simulink model "MUTfinal2"  (R2022b)
settings: Solver=VariableStepAuto  StartTime=0.0  StopTime=tFinal  RelTol=1e-3
values from neighbouring files (symbols this model uses):
  C1 = C1_OLD    [DPP_PSO.m]    (also in PlotEvaluateResponse.m = 1.59e-06)
  C2 = C2_OLD    [DPP_PSO.m]    (also in PlotEvaluateResponse.m = 1.59e-06)
  Cn = Cn_OLD    [DPP_PSO.m]    (also in PlotEvaluateResponse.m = 7.95e-07)
  F = 20e3    (= 20000)    [DPP_PSO.m]    (also in PlotEvaluateResponse.m)
  G1 = 1000    [DPP_PSO.m]    (also in PlotEvaluateResponse.m)
  L1 = L1_OLD    [DPP_PSO.m]    (also in PlotEvaluateResponse.m = 0.0049)
  L2 = L2_OLD    [DPP_PSO.m]    (also in PlotEvaluateResponse.m = 0.0049)
  sample_time = 1e-6    (= 1e-06)    [DPP_PSO.m]    (also in PlotEvaluateResponse.m)
  VBus = 36    [DPP_PSO.m]    (also in PlotEvaluateResponse.m)
undefined symbols (not defined in the file or in its folder): sigbuilder_block
libraries: spsSeriesRLCBranchLib x6, spsCurrentMeasurementLib x6, spsVoltageMeasurementLib x4, spsDiodeLib x2, spsPVArrayLib x2, spsMosfetLib x2, spsDCVoltageSourceLib x1, spspowerguiLib x1
settings Model: Creator=gta12345_v  LastModifiedBy=AEssa
settings ModelReferenceCC: EnableRefExpFcnMdlSchedulingChecks=on

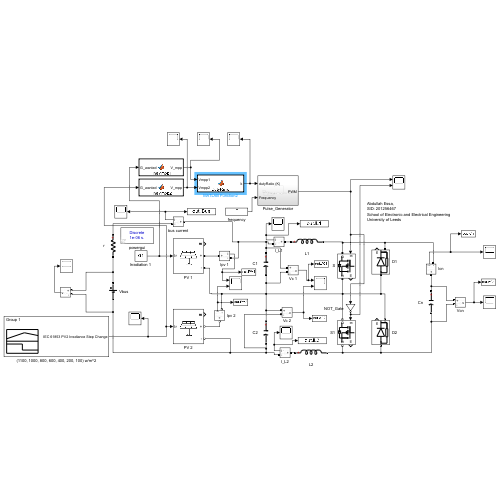
[thumbnail: Simulink's stored preview of the top-level diagram]
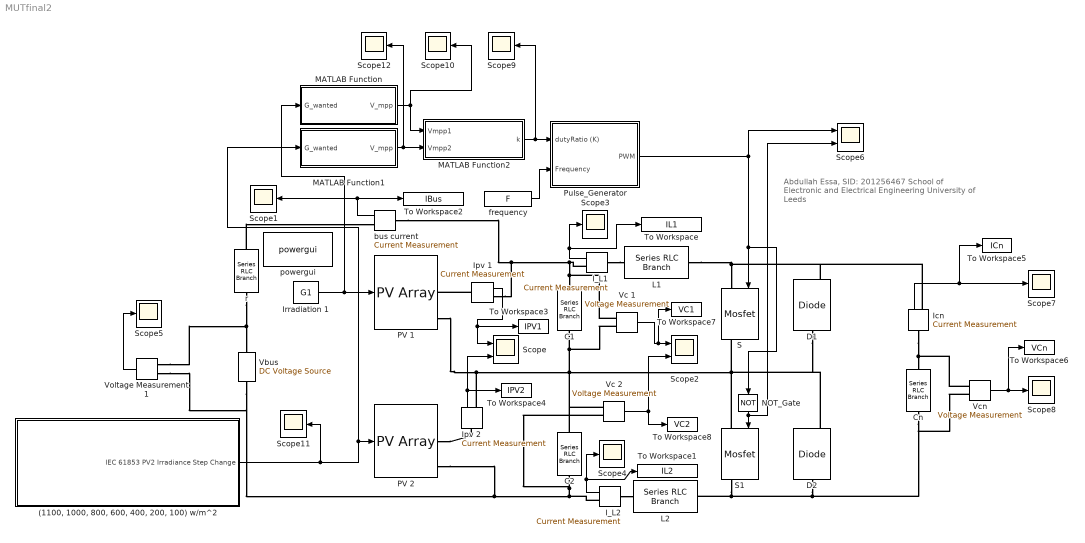
== system MUTfinal2 ==
  note: Abdullah Essa,
      | SID: 201256467
      | School of Electronic and Electrical Engineering
      | University of Leeds
  "(1100, 1000, 800, 600, 400, 200, 100) w/m^2" : Subsystem  Tag=STV Subsys  LoadFcn=sigbuilder_block('load');  StartFcn=sigbuilder_block('start');  StopFcn=sigbuilder_block('stop');  ClipboardFcn=sigbuilder_block('clipboard');  mask(Sigbuilder block){tuvar=[0:10]}
      mask help: Simulink:masks:SigbuilderBlock_MD
      mask init:
      | if ~strcmp(get_param(bdroot(gcbh),'SimulationStatus'),'stopped') tuvar = sigbuilder_block('maskInit'); end
      settings: CopyFcn=sigbuilder_block('copy');  DeleteFcn=sigbuilder_block('delete');  ModelCloseFcn=sigbuilder_block('modelClose');  PreSaveFcn=sigbuilder_block('preSave');  PauseFcn=sigbuilder_block('pause');  ContinueFcn=sigbuilder_block('continue');  NameChangeFcn=sigbuilder_block('namechange');  OpenFcn=sigbuilder_block('open',[420 17.25 550.5 399.75 ]);  CloseFcn=sigbuilder_block('close');
      mask Display: plot(0, 0, 100, 100,[2, 2, 32, 32, 2], [68, 8, 8, 68, 68],[32, 2], [38, 38], [32, 19, 2],[53, 60, 44], [32, 17, 17, 2],[16, 16, 31, 31]);txt = getActiveGroup(gcbh);text(2, 100, txt,'verticalAlignment', 'top');
  C1 : spsSeriesRLCBranchLib/Series RLC Branch  LConnTagsString=__new0  RConnTagsString=__new0  BranchType=C  Resistance=1  Inductance=1e-3  SetiL0=off  InitialCurrent=0  Capacitance=C1  Setx0=off  InitialVoltage=0  Measurements=None
  C2 : spsSeriesRLCBranchLib/Series RLC Branch  LConnTagsString=__new0  RConnTagsString=__new0  BranchType=C  Resistance=1  Inductance=1e-3  SetiL0=off  InitialCurrent=0  Capacitance=C2  Setx0=off  InitialVoltage=0  Measurements=None
  Cn : spsSeriesRLCBranchLib/Series RLC Branch  LConnTagsString=__new0  RConnTagsString=__new0  BranchType=C  Resistance=1  Inductance=1e-3  SetiL0=off  InitialCurrent=0  Capacitance=Cn  Setx0=off  InitialVoltage=0  Measurements=None
  D1 : spsDiodeLib/Diode  Ron=0.001  Lon=0  Vf=0.8  IC=0  UseSnubber=0  Rs=500  Cs=250e-9  Measurements=on
  D2 : spsDiodeLib/Diode  Ron=0.001  Lon=0  Vf=0.8  IC=0  UseSnubber=0  Rs=500  Cs=250e-9  Measurements=on
  I_L1 : spsCurrentMeasurementLib/Current Measurement  PhasorSimulation=off  OutputType=Complex  PSBequivalent=0
  I_L2 : spsCurrentMeasurementLib/Current Measurement  PhasorSimulation=off  OutputType=Complex  PSBequivalent=0
  "Icn " : spsCurrentMeasurementLib/Current Measurement  PhasorSimulation=off  OutputType=Complex  PSBequivalent=0
  Ipv 1 : spsCurrentMeasurementLib/Current Measurement  PhasorSimulation=off  OutputType=Complex  PSBequivalent=0
  Ipv 2 : spsCurrentMeasurementLib/Current Measurement  PhasorSimulation=off  OutputType=Complex  PSBequivalent=0
  "Irradiation 1 " : Constant  Value=G1  SampleTime=Inf
  L1 : spsSeriesRLCBranchLib/Series RLC Branch  LConnTagsString=__new0  RConnTagsString=__new0  BranchType=L  Resistance=1  Inductance=L1  SetiL0=off  InitialCurrent=0  Capacitance=1e-6  Setx0=off  InitialVoltage=0  Measurements=None
  L2 : spsSeriesRLCBranchLib/Series RLC Branch  LConnTagsString=__new0  RConnTagsString=__new0  BranchType=L  Resistance=1  Inductance=L2  SetiL0=off  InitialCurrent=0  Capacitance=1e-6  Setx0=off  InitialVoltage=0  Measurements=None
  MATLAB Function : MATLAB Function  TreatAsAtomicUnit=on
  MATLAB Function1 : MATLAB Function  TreatAsAtomicUnit=on
  MATLAB Function2 : MATLAB Function  TreatAsAtomicUnit=on
  NOT_Gate : Logic  Operator=NOT  IconShape=distinctive  AllPortsSameDT=off  OutDataTypeStr=boolean
  PV 1 : spsPVArrayLib/PV Array  Npar=1  Nser=1  PlotType=one module @ 25 deg.C & specified irradiances  S_vec="[ 1000  500  100 ]"  Temp_C_vec="[ 45 25  ]"  ModuleName=Canadian Solar Inc. CS5C-90M  PlotWhenSelected=off  Pm=89.82  Ncell=36  Voc=22.2  Isc=5.4  Vm=18  Im=4.99  beta_Voc_pc=-0.374  alpha_Isc_pc=0.089  beta_Voc=-0.083028  alpha_Isc=0.004806  IL=5.4115  I0=3.0531e-10  nI=1.0185  Rsh=134.0722  Rs=0.2862  RobustModel=on  RobustCellTemperature=25  BAL=on  Tc=1e-6  Tfilter=5e-5
  PV 2 : spsPVArrayLib/PV Array  Npar=1  Nser=1  PlotType=one module @ 25 deg.C & specified irradiances  S_vec="[ 1000  500  100 ]"  Temp_C_vec="[ 45 25  ]"  ModuleName=Canadian Solar Inc. CS5C-90M  PlotWhenSelected=off  Pm=89.82  Ncell=36  Voc=22.2  Isc=5.4  Vm=18  Im=4.99  beta_Voc_pc=-0.374  alpha_Isc_pc=0.089  beta_Voc=-0.083028  alpha_Isc=0.004806  IL=5.4115  I0=3.0531e-10  nI=1.0185  Rsh=134.0722  Rs=0.2862  RobustModel=on  RobustCellTemperature=25  BAL=on  Tc=1e-6  Tfilter=5e-5
  Pulse_Generator : Subsystem
  S : spsMosfetLib/Mosfet  Ron=0.1  Lon=0  Rd=0.01  Vfd=0  IC=0  Rs=1e5  Cs=inf  Measurements=on
  S1 : spsMosfetLib/Mosfet  Ron=0.1  Lon=0  Rd=0.01  Vfd=0  IC=0  Rs=1e5  Cs=inf  Measurements=on
  Scope : Scope  NumInputPorts=2
  Scope{1,3..5,7..12} (10 alike) : Scope
  Scope2 : Scope  NumInputPorts=2
  Scope6 : Scope  NumInputPorts=2
  To Workspace : ToWorkspace  VariableName=IL1  SaveFormat=Timeseries  SampleTime=-1
  To Workspace1 : ToWorkspace  VariableName=IL2  SaveFormat=Timeseries  SampleTime=-1
  To Workspace2 : ToWorkspace  VariableName=IBus  SaveFormat=Timeseries  SampleTime=-1
  To Workspace3 : ToWorkspace  VariableName=IPV1  SaveFormat=Timeseries  SampleTime=-1
  To Workspace4 : ToWorkspace  VariableName=IPV2  SaveFormat=Timeseries  SampleTime=-1
  To Workspace5 : ToWorkspace  VariableName=ICn  SaveFormat=Timeseries  SampleTime=-1
  To Workspace6 : ToWorkspace  VariableName=VCn  SaveFormat=Timeseries  SampleTime=-1
  To Workspace7 : ToWorkspace  VariableName=VC1  SaveFormat=Timeseries  SampleTime=-1
  To Workspace8 : ToWorkspace  VariableName=VC2  SaveFormat=Timeseries  SampleTime=-1
  Vbus : spsDCVoltageSourceLib/DC Voltage Source  Amplitude=VBus  Measurements=None
  Vc 1 : spsVoltageMeasurementLib/Voltage Measurement  PhasorSimulation=off  OutputType=Complex  PSBequivalent=0
  Vc 2 : spsVoltageMeasurementLib/Voltage Measurement  PhasorSimulation=off  OutputType=Complex  PSBequivalent=0
  Vcn : spsVoltageMeasurementLib/Voltage Measurement  PhasorSimulation=off  OutputType=Complex  PSBequivalent=0
  Voltage Measurement1 : spsVoltageMeasurementLib/Voltage Measurement  PhasorSimulation=off  OutputType=Complex  PSBequivalent=0
  bus current : spsCurrentMeasurementLib/Current Measurement  PhasorSimulation=off  OutputType=Complex  PSBequivalent=0
  frequency : Constant  Value=F
  powergui : spspowerguiLib/powergui  Priority=1  SimulationMode=Discrete  SampleTime=sample_time  frequency=60  Iterations=50  frequencyindice=0  Pbase=100e6  ErrMax=1e-4  UnitsV=kV  UnitsW=MW  buscounter=0  FunctionMessages=off  echomessages=off  EnableUseOfTLC=off  CurrentSourceSwitches=off  DisableSnubberDevices=off  DisableRonSwitches=off  DisableVfSwitches=off  DisplayEquations=off  AutomaticDiscreteSolvers=off  SolverType=Tustin/Backward Euler (TBE)  Interpol=off  ExternalGateDelay=off  methode=off  Ts=100  x0status=blocks  SPID=on  SwTol=0  HookPort=off  NonlinearTolerance=1e-4  nMaxIteration=100  ContinueOnMaxIteration=off  RestoreLinks=warning  ResistiveCurrentMeasurement=off  Frange=[0:2:500]  Ylog=off  Xlog=on  ShowGrid=off  save=off  variable=ZData  structure=0  ZoomFFT=off  StartTime=0.0  cycles=1  DisplayStyle=1  fundamental=60  FreqAxis=off  MaxFrequency=1000  frequencyindicesteady=1  RmsSteady=1  display=off
  r : spsSeriesRLCBranchLib/Series RLC Branch  LConnTagsString=__new0  RConnTagsString=__new0  BranchType=R  Resistance=0.1  Inductance=1e-3  SetiL0=off  InitialCurrent=0  Capacitance=1.59e-6  Setx0=off  InitialVoltage=0  Measurements=None
  wires:
  "Irradiation 1 "/1 -> MATLAB Function/1(G_wanted), PV 1/1
  Pulse_Generator/1(PWM) -> Scope6/1, NOT_Gate/1, S/1
  NOT_Gate/1 -> Scope6/2, S1/1
  Ipv 2/1 -> To Workspace4/1, Scope/2
  Ipv 1/1 -> To Workspace3/1, Scope/1
  bus current/1 -> To Workspace2/1, Scope1/1
  Vc 1/1 -> To Workspace7/1, Scope2/1
  I_L2/1 -> Scope4/1, To Workspace1/1
  I_L1/1 -> To Workspace/1, Scope3/1
  Voltage Measurement1/1 -> Scope5/1
  "(1100, 1000, 800, 600, 400, 200, 100) w/m^2"/1(IEC 61853 PV2 Irradiance Step Change) -> Scope11/1, MATLAB Function1/1(G_wanted), PV 2/1
  frequency/1 -> Pulse_Generator/2(Frequency)
  Vc 2/1 -> To Workspace8/1, Scope2/2
  "Icn "/1 -> To Workspace5/1, Scope7/1
  Vcn/1 -> To Workspace6/1, Scope8/1
  MATLAB Function/1(V_mpp) -> MATLAB Function2/1(Vmpp1), Scope10/1
  MATLAB Function1/1(V_mpp) -> Scope12/1, MATLAB Function2/2(Vmpp2)
  MATLAB Function2/1(k) -> Scope9/1, Pulse_Generator/1(dutyRatio (K))
  connections:
  bus current/LConn1 -- Ipv 1/RConn1 -- Vc 1/LConn1 -- C1/LConn1 -- I_L1/RConn1
  PV 2/RConn2 -- Vbus/LConn1 -- Voltage Measurement1/LConn2 -- I_L2/RConn1 -- Vc 2/LConn2 -- C2/RConn1
  L1/RConn1 -- "Icn "/RConn1 -- D1/RConn1 -- S/LConn1
  PV 1/RConn2 -- Ipv 2/RConn1 -- Vc 2/LConn1 -- C2/LConn1 -- Vc 1/LConn2 -- C1/RConn1 -- D2/RConn1 -- D1/LConn1 -- S/RConn1 -- S1/LConn1
  S1/RConn1 -- Vcn/LConn2 -- Cn/RConn1 -- D2/LConn1 -- L2/RConn1
  Voltage Measurement1/LConn1 -- r/RConn1 -- Vbus/RConn1
  Ipv 1/LConn1 -- PV 1/RConn1
  PV 2/RConn1 -- Ipv 2/LConn1
  I_L1/LConn1 -- L1/LConn1
  I_L2/LConn1 -- L2/LConn1
  r/LConn1 -- bus current/RConn1
  "Icn "/LConn1 -- Vcn/LConn1 -- Cn/LConn1

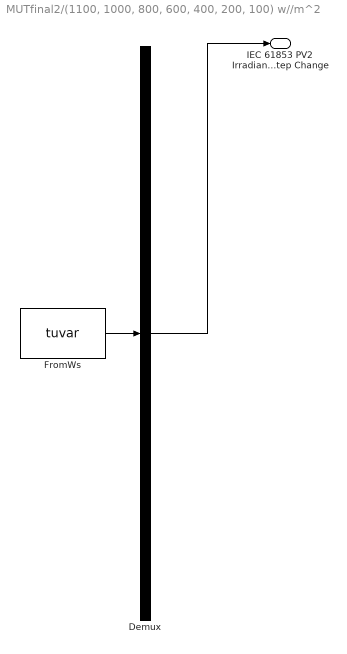
== system MUTfinal2/(1100, 1000, 800, 600, 400, 200, 100) w//m^2 ==
  Demux : Demux  Tag=STV Demux  Outputs=1
      settings: DisplayOption=none
  FromWs : FromWorkspace  Tag=STV FromWs  VariableName=tuvar
      SigBuilderData=|
      | common.afterFinalStr = 'Extrapolate'
      | common.sampleTime = 0
      | dataSet.timeRange = [0 0.14]
      | dataSet.name = 'Group 1'
      | sbobj.Groups.Name = 'Group 1'
      | sbobj.Groups.Signals.Name = 'IEC 61853 PV2 Irradiance Step Change'
      | sbobj.Groups.Signals.XData = [0 0.02 0.02 0.04 0.04 0.06 0.06 0.08 0.08 0.1 0.1 0.12 0.12 0.14]
      | sbobj.Groups.Signals.YData = [1100 1100 1000 1000 800 800 600 600 400 400 200 200 100 100]
      | sbobj.Groups.TimeRange = [0 0.14]
  IEC 61853 PV2 Irradiance Step Change : Outport  Tag=STV Outport
  wires:
  Demux/1 -> IEC 61853 PV2 Irradiance Step Change/1
  FromWs/1 -> Demux/1

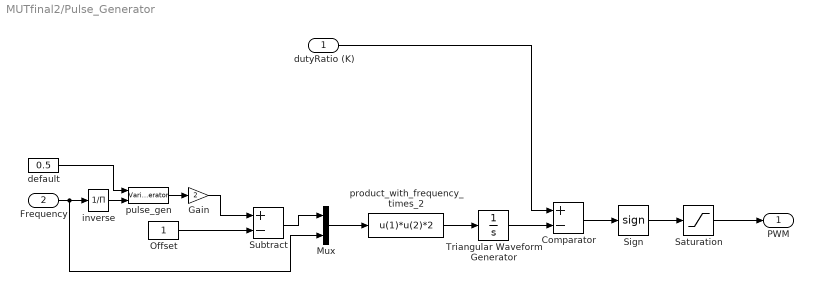
== system MUTfinal2/Pulse_Generator ==
  dutyRatio (K) : Inport
  Frequency : Inport  Port=2
  Comparator : Sum  Inputs=+-
  Gain : Gain  Gain=2
  Mux : Mux  Inputs=2
  Offset : Constant
  Saturation : Saturate  UpperLimit=1  LowerLimit=0
  Sign : Signum
  Subtract : Sum  Inputs=+-
  Triangular Waveform Generator : Integrator
  default : Constant  Value=0.5
  inverse : Product  Inputs=/
  product_with_frequency_times_2 : Fcn  Expr=u(1)*u(2)*2
  pulse_gen : VariablePulseGenerator  SampleTime=0.1
  PWM : Outport
  wires:
  Subtract/1 -> Mux/1
  Sign/1 -> Saturation/1
  Triangular Waveform Generator/1 -> Comparator/2
  Offset/1 -> Subtract/2
  Comparator/1 -> Sign/1
  dutyRatio (K)/1 -> Comparator/1
  Saturation/1 -> PWM/1
  Frequency/1 -> Mux/2, inverse/1
  inverse/1 -> pulse_gen/2
  pulse_gen/1 -> Gain/1
  default/1 -> pulse_gen/1
  Mux/1 -> product_with_frequency_times_2/1
  product_with_frequency_times_2/1 -> Triangular Waveform Generator/1
  Gain/1 -> Subtract/1

== matlab function MUTfinal2/MATLAB Function ==
  data: G_wanted input; V_mpp output
function V_mpp = FindVmpp1(G_wanted)

G_wanted1 = G_wanted;
V_wanted1 = 0;
V_point1 = 0;
V_point2 = 0;
G_point1 = 0;
G_point2 = 0;

% IEC 61853 irradiance values 
G = [100, 200, 400, 600, 800, 1000, 1100];

% Corresponding mpp voltages 
Vmpp = [17.08, 17.61, 17.94, 18.06, 18.04, 18, 17.97];

% deducing mpp voltage
for i = (2:length(G))

    if (G_wanted1 == G(i))  
        V_wanted1 = Vmpp(i);
        break;

    elseif (G_wanted1 == G(i-1)) 
        V_wanted1 = Vmpp(i-1);
        break;

    elseif (G_wanted1 < G(1))

        V_point1 = 0;
        V_point2 = Vmpp(length(Vmpp));
        G_point1 = 0;
        G_point2 = min(G);
        
        Gradient1 = (V_point2 - V_point1)/(G_point2 - G_point1);
        V_wanted1 = V_point1 + Gradient1*(G_wanted1 - G_point1);
        break;

    elseif (G_wanted1 > G(length(G)))

        V_wanted1 = Vmpp(i);  % cannot find unknown gradient

    elseif (G_wanted1 < G(i) && G_wanted1 > G(i-1))
        % for when the data point is between to known points
        V_point1 = Vmpp(i-1);
        V_point2 = Vmpp(i);
        G_point1 = G(i-1);
        G_point2 =  G(i);
        
        Gradient1 = (V_point2 - V_point1)/(G_point2 - G_point1);
        V_wanted1 = V_point1 + Gradient1*(G_wanted1 - G_point1);
    end
end

% output result
V_mpp = V_wanted1;

== matlab function MUTfinal2/MATLAB Function2 ==
  data: Vmpp1 input; k output; Vmpp2 input
function k = DutyRatio(Vmpp1, Vmpp2)

k = Vmpp2/(Vmpp2+Vmpp1);

== matlab function MUTfinal2/MATLAB Function1 ==
  data: G_wanted input; V_mpp output
function V_mpp = FindVmpp2(G_wanted)

G_wanted1 = G_wanted;
V_wanted1 = 0;
V_point1 = 0;
V_point2 = 0;
G_point1 = 0;
G_point2 = 0;

% IEC 61853 irradiance values 
G = [100, 200, 400, 600, 800, 1000, 1100];

% Corresponding mpp voltages 
Vmpp = [17.08, 17.61, 17.94, 18.06, 18.04, 18, 17.97];

% deducing mpp voltage
for i = (2:length(G))

    if (G_wanted1 == G(i))  
        V_wanted1 = Vmpp(i);
        break;

    elseif (G_wanted1 == G(i-1)) 
        V_wanted1 = Vmpp(i-1);
        break;

    elseif (G_wanted1 < G(1))

        V_point1 = 0;
        V_point2 = Vmpp(length(Vmpp));
        G_point1 = 0;
        G_point2 = min(G);
        
        Gradient1 = (V_point2 - V_point1)/(G_point2 - G_point1);
        V_wanted1 = V_point1 + Gradient1*(G_wanted1 - G_point1);
        break;

    elseif (G_wanted1 > G(length(G)))

        V_wanted1 = Vmpp(i);  % cannot find unknown gradient

    elseif (G_wanted1 < G(i) && G_wanted1 > G(i-1))
        % for when the data point is between to known points
        V_point1 = Vmpp(i-1);
        V_point2 = Vmpp(i);
        G_point1 = G(i-1);
        G_point2 =  G(i);
        
        Gradient1 = (V_point2 - V_point1)/(G_point2 - G_point1);
        V_wanted1 = V_point1 + Gradient1*(G_wanted1 - G_point1);
    end
end

% output result
V_mpp = V_wanted1;
